simulink model "slexMicrophoneBeamformerExample"  (R2024b)
settings: Solver=FixedStepDiscrete  StartTime=0.0  StopTime=inf  RelTol=1e-3  EnableMultiTasking=on
undefined symbols (not defined in the file or in its folder): phased
libraries: dspvision x3, phasedtxrxlib x2, dspsnks4 x1, phasedbflib x1, phasedmisclib x1
Description:
  | Acoustic Beamforming using Microphone Arrays
settings Model: Creator=The MathWorks, Inc.  LastModifiedBy=The MathWorks, Inc.
settings SolverCC: AlgebraicLoopSolver=TrustRegion
settings DataIOCC: LimitDataPoints=on  SaveFormat=Array  ReturnWorkspaceOutputs=off
settings OptimizationCC: LifeSpan=inf
settings DebuggingCC: ReadBeforeWriteMsg=DisableAll  WriteAfterWriteMsg=DisableAll  WriteAfterReadMsg=DisableAll  UnderspecifiedInitializationDetection=Classic  MergeDetectMultiDrivingBlocksExec=none  SolverPrmCheckMsg=warning  UnconnectedInputMsg=warning  UnconnectedOutputMsg=warning  UnconnectedLineMsg=warning  AllowSymbolicDim=off  SFUnexpectedBacktrackingDiag=warning  SFNoUnconditionalDefaultTransitionDiag=warning  SFExecutionAtInitializationDiag=none  ArithmeticOperatorsInVariantConditions=warning
settings HardwareCC: ProdBitPerPointer=32  ProdBitPerSizeT=32  ProdBitPerPtrDiffT=32  ProdLargestAtomicFloat=None  ProdIntDivRoundTo=Undefined  ProdEndianess=Unspecified  ProdWordSize=32  ProdHWDeviceType=32-bit Generic
settings ModelReferenceCC: EnableRefExpFcnMdlSchedulingChecks=on  PropagateSignalLabelsOutOfModel=off
settings SFSimCC: SimUseLocalCustomCode=off  CustomCodeUndefinedFunction=UseInterfaceOnly
settings RTWCC: RTWUseLocalCustomCode=off  GPUComputeCapability=3.5
settings CodeAppCC: StateflowObjectComments=on
settings GRTTargetCC: TargetLangStandard=C89/C90 (ANSI)
settings ConfigComp: CovMetricSettings=dw  CovSaveCumulativeToWorkspaceVar=on  CovSaveSingleToWorkspaceVar=on  CovExternalEMLEnable=off  CovSFcnEnable=off

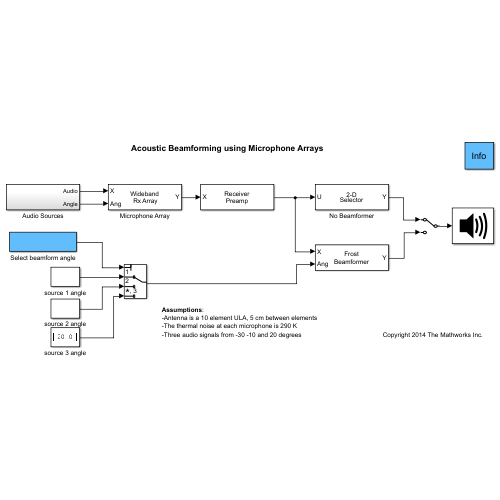
[thumbnail: Simulink's stored preview of the top-level diagram]
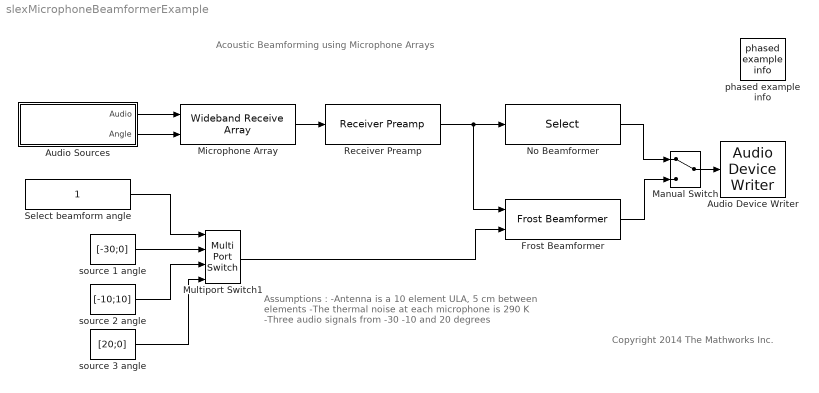
== system slexMicrophoneBeamformerExample ==
  note: Acoustic Beamforming using Microphone Arrays
  note: Assumptions :
      | -Antenna is a 10 element ULA, 5 cm between elements
      | -The thermal noise at each microphone is 290 K
      | -Three audio signals from -30 -10 and 20 degrees
  note: Copyright 2014 The Mathworks Inc.
  Audio Device Writer : dspsnks4/Audio Device Writer  Driver=DirectSound  Device=Default  InheritSampleRate=on  SampleRate=44100  BitDepth=16-bit integer  BufferSize=4096  NumBuffers=10  DefaultOutputChannelMapping=on  OutputChannelMapping=1:2  OutputNumUnderrunSamples=off  DriverIdx=1  DeviceWarnFlag=''
  Audio Sources : Subsystem
  Frost Beamformer : phasedbflib/Frost Beamformer  PropagationSpeed=340  SampleRateFromInputCheckbox=on  SampleRate=1e6  FilterLength=20  DiagonalLoadingFactor=0  TrainingInputPort=off  DirectionSource=Input port  Direction=[ 0; 0 ]  WeightsOutputPort=off  SimulateUsing=Interpreted execution  SensorArray=phased.ULA('Element',phased.OmnidirectionalMicrophoneElement(),'NumElements',10,'ElementSpacing',0.05)
  Manual Switch : ManualSwitch
  Microphone Array : phasedtxrxlib/Wideband Receive Array  PropagationSpeed=340  SampleRateFromInputCheckbox=on  SampleRate=1e6  ModulatedInput=off  CarrierFrequency=1e9  NumSubbands=64  Wavefront=Plane  SensorGainMeasure=dB  Polarization=None  WeightsInputPort=off  SimulateUsing=Interpreted execution  Sensor=phased.ULA('Element',phased.OmnidirectionalMicrophoneElement(),'NumElements',10,'ElementSpacing',0.05)
  Multiport Switch1 : MultiPortSwitch  SaturateOnIntegerOverflow=off  InputSameDT=off
  No Beamformer : Selector  NumberOfDimensions=2  InputPortWidth=3  IndexOptions=Select all,Index vector (dialog)  Indices=[1 3],5  OutputSizes=1,1
  Receiver Preamp : phasedtxrxlib/Receiver Preamp  Gain=0  LossFactor=0  NoiseMethod=Noise temperature  NoiseFigure=0  ReferenceTemperature=290  SampleRateFromInputCheckbox=on  SampleRate=1e6  NoisePower=0  EnableInputPort=off  PhaseNoiseInputPort=off  SeedSource=Auto  Seed=0  SimulateUsing=Interpreted execution
  Select beamform angle : Constant
  phased example info : phasedmisclib/phased example info  SystemSampleTime=-1  VariantActivationTime=update diagram  AllowFlexibleInterface=on  Latency=0  AutoFrameSizeCalculation=off
  source 1 angle : Constant  Value=[-30;0]
  source 2 angle : Constant  Value=[-10;10]
  source 3 angle : Constant  Value=[20;0]
  wires:
  Frost Beamformer/1 -> Manual Switch/2
  Multiport Switch1/1 -> Frost Beamformer/2
  Manual Switch/1 -> Audio Device Writer/1
  source 1 angle/1 -> Multiport Switch1/2
  source 2 angle/1 -> Multiport Switch1/3
  source 3 angle/1 -> Multiport Switch1/4
  Select beamform angle/1 -> Multiport Switch1/1
  Audio Sources/1(Audio) -> Microphone Array/1
  No Beamformer/1 -> Manual Switch/1
  Receiver Preamp/1 -> Frost Beamformer/1, No Beamformer/1
  Microphone Array/1 -> Receiver Preamp/1
  Audio Sources/2(Angle) -> Microphone Array/2

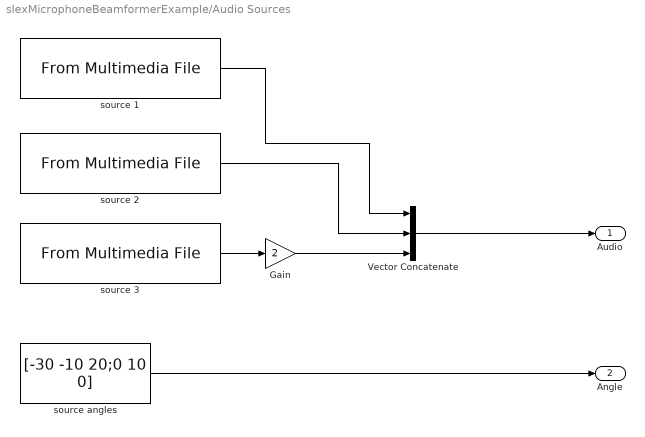
== system slexMicrophoneBeamformerExample/Audio Sources ==
  Gain : Gain  Gain=2
  Vector Concatenate : Concatenate  NumInputs=3  Mode=Multidimensional array  ConcatenateDimension=2
  source 1 : dspvision/From Multimedia File  inputFilename=dft_voice_8kHz.wav  readRange=[1 Inf]  loop=on  numPlays=inf  outputStreams=Audio only  videoDataType=single  audioDataType=double  inheritSampleTime=on  userDefinedSampleTime=1/30  noAudioOutput=off  isIntensityVideo=off  fourcc=RGB  colorVideoFormat=Separate color signals  outputEOF=off  dataOrg=Column-major  audioFrameSize=1000  computeAudioFrameSize=off  outSamplingMode=Sample based
  source 2 : dspvision/From Multimedia File  inputFilename=cleanspeech_voice_8kHz.wav  readRange=[1 Inf]  loop=on  numPlays=inf  outputStreams=Audio only  videoDataType=single  audioDataType=double  inheritSampleTime=on  userDefinedSampleTime=1/30  noAudioOutput=off  isIntensityVideo=off  fourcc=RGB  colorVideoFormat=Separate color signals  outputEOF=off  dataOrg=Column-major  audioFrameSize=1000  computeAudioFrameSize=off  outSamplingMode=Sample based
  source 3 : dspvision/From Multimedia File  inputFilename=laughter_8kHz.wav  readRange=[1 Inf]  loop=on  numPlays=inf  outputStreams=Audio only  videoDataType=single  audioDataType=double  inheritSampleTime=on  userDefinedSampleTime=1/30  noAudioOutput=off  isIntensityVideo=off  fourcc=RGB  colorVideoFormat=Separate color signals  outputEOF=off  dataOrg=Column-major  audioFrameSize=1000  computeAudioFrameSize=off  outSamplingMode=Sample based
  source angles : Constant  Value=[-30 -10 20;0 10 0]
  Audio : Outport  VectorParamsAs1DForOutWhenUnconnected=off
  Angle : Outport  Port=2  VectorParamsAs1DForOutWhenUnconnected=off
  wires:
  source 1/1 -> Vector Concatenate/1
  source 3/1 -> Gain/1
  source 2/1 -> Vector Concatenate/2
  Gain/1 -> Vector Concatenate/3
  Vector Concatenate/1 -> Audio/1
  source angles/1 -> Angle/1
